simulink model "tanhModAmpModu"  (R2022a)
settings: Solver=VariableStepAuto  StartTime=0.0  StopTime=50  RelTol=1e-3
values from neighbouring files (symbols this model uses):
  bar_amp = 0.4    [setup_runAmpModu.m]
  delta_gsm = -0.025    [setup_runAmpModu.m]
  dfm1 = 0.0    (= 0)    [setup_run.m]    (also in setup_runAmpModu.m)
  dfm1s = 0.0    (= 0)    [setup_runAmpModu.m]
  dfm2 = 0.0    (= 0)    [setup_run.m]    (also in setup_runAmpModu.m)
  dsm1 = -0.5    [setup_run.m]    (also in setup_runAmpModu.m)
  dsm1s = -0.5    [setup_runAmpModu.m]
  dsm2 = -0.5    [setup_run.m]    (also in setup_runAmpModu.m)
  dsp1 = 0.5    [setup_run.m]    (also in setup_runAmpModu.m)
  dsp1s = 0.5    [setup_runAmpModu.m]
  dsp2 = 0.5    [setup_run.m]    (also in setup_runAmpModu.m)
  dup1 = -0.5    [setup_run.m]    (also in setup_runAmpModu.m)
  dup1s = -0.5    [setup_runAmpModu.m]
  dup2 = -0.5    [setup_run.m]    (also in setup_runAmpModu.m)
  gfm1 = -2.0+0.01    (= -1.99)    [setup_run.m]    (also in setup_runAmpModu.m)
  gfm1s = -2.0+0.01    (= -1.99)    [setup_runAmpModu.m]
  gfm2 = -2.0-0.01    (= -2.01)    [setup_run.m]    (also in setup_runAmpModu.m)
  gsm0 = -3.0    (= -3)    [setup_runAmpModu.m]
  gsm1s = -1.0+0.01    (= -0.99)    [setup_runAmpModu.m]
  gsp1 = 6.0-0.01    (= 5.99)    [setup_run.m]    (also in setup_runAmpModu.m = 6.99)
  gsp1s = 4.0-0.01    (= 3.99)    [setup_runAmpModu.m]
  gsp2 = 6.0+0.01    (= 6.01)    [setup_run.m]    (also in setup_runAmpModu.m = 7.01)
  gsyn12 = -0.2    [setup_run.m]    (also in setup_runAmpModu.m)
  gsyn21 = -0.2    [setup_run.m]    (also in setup_runAmpModu.m)
  gup1 = 5.0-0.01    (= 4.99)    [setup_run.m]    (also in setup_runAmpModu.m)
  gup1s = 1.0-0.01    (= 0.99)    [setup_runAmpModu.m]
  gup2 = 5.0+0.01    (= 5.01)    [setup_run.m]    (also in setup_runAmpModu.m)
  Iapp1 = -1.0    (= -1)    [setup_run.m]    (also in setup_runAmpModu.m = -1.05)
  Iapp1s = -0.05    [setup_runAmpModu.m]
  Iapp2 = -1.0    (= -1)    [setup_run.m]    (also in setup_runAmpModu.m = -0.95)
  max_torque = 10.0    (= 10)    [setup_run.m]    (also in setup_runAmpModu.m)
  noise_pwr = 0.0    (= 0)    [setup_runAmpModu.m]
  rflx_g = 0.0    (= 0)    [setup_run.m]    (also in setup_runAmpModu.m = 0.1)
undefined symbols (not defined in the file or in its folder): X, Y, Z
libraries: sm_lib x6, nesl_utility x3, simulink x3
settings Model: Creator=alessiofranci  LastModifiedBy=chris

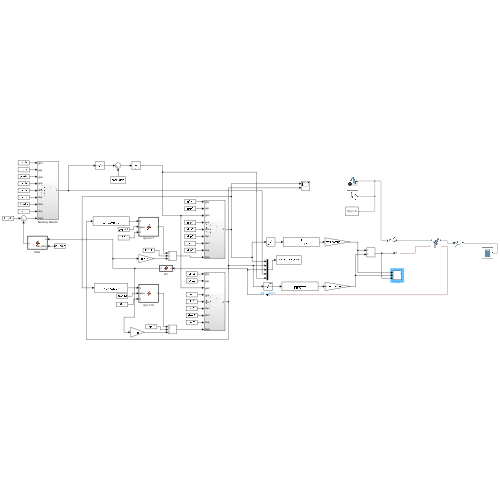
[thumbnail: Simulink's stored preview of the top-level diagram]
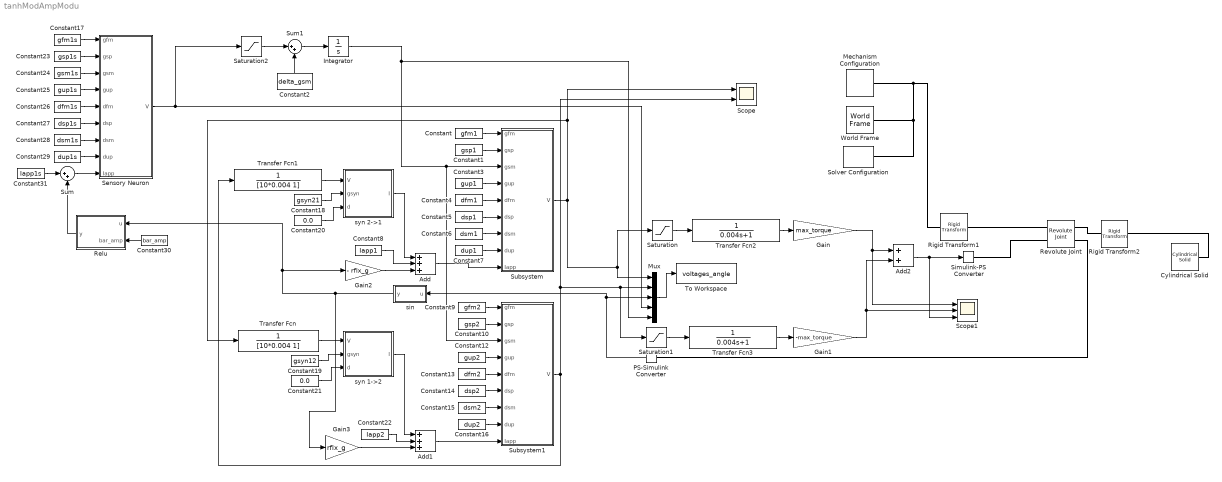
== system tanhModAmpModu ==
  Add : Sum  Inputs=+++
  Add1 : Sum  Inputs=+++
  Add2 : Sum
  Constant : Constant  Value=gfm1
  Constant1 : Constant  Value=gsp1
  Constant10 : Constant  Value=gsp2
  Constant12 : Constant  Value=gup2
  Constant13 : Constant  Value=dfm2
  Constant14 : Constant  Value=dsp2
  Constant15 : Constant  Value=dsm2
  Constant16 : Constant  Value=dup2
  Constant17 : Constant  Value=gfm1s
  Constant18 : Constant  Value=gsyn21
  Constant19 : Constant  Value=gsyn12
  Constant2 : Constant  Value=delta_gsm
  Constant20 : Constant  Value=0.0
  Constant21 : Constant  Value=0.0
  Constant22 : Constant  Value=Iapp2
  Constant23 : Constant  Value=gsp1s
  Constant24 : Constant  Value=gsm1s
  Constant25 : Constant  Value=gup1s
  Constant26 : Constant  Value=dfm1s
  Constant27 : Constant  Value=dsp1s
  Constant28 : Constant  Value=dsm1s
  Constant29 : Constant  Value=dup1s
  Constant3 : Constant  Value=gup1
  Constant30 : Constant  Value=bar_amp
  Constant31 : Constant  Value=Iapp1s
  Constant4 : Constant  Value=dfm1
  Constant5 : Constant  Value=dsp1
  Constant6 : Constant  Value=dsm1
  Constant7 : Constant  Value=dup1
  Constant8 : Constant  Value=Iapp1
  Constant9 : Constant  Value=gfm2
  Cylindrical Solid : sm_lib/Body Elements/Cylindrical Solid  GraphicAmbientColor=[0.15 0.15 0.15 1.0]  BasedOnType=Density  CenterOfMass=[0 0 0]  CenterOfMassUnits=m  GraphicDiffuseColor=[0.5 0.5 0.5]  CylinderLength=bar_length  CylinderLengthUnits=m  CylinderRadius=0.05  CylinderRadiusUnits=m  Density=1000  DensityUnits=kg/m^3  DoExposeReferenceFrame=on  GraphicEmissiveColor=[0.0 0.0 0.0 1.0]  ExportEntireGeometry=off  SerializedFrames=<Frames/>  MarkerShape=Sphere  MarkerSize=10  GraphicType=FromGeometry  InertiaType=CalculateFromGeometry  Mass=1  MassUnits=kg  MomentsOfInertia=[1 1 1]  MomentsOfInertiaUnits=kg*m^2  GraphicOpacity=1.0  ProductsOfInertia=[0 0 0]  ProductsOfInertiaUnits=kg*m^2  GraphicShininess=75  GraphicSpecularColor=[0.5 0.5 0.5 1.0]  GraphicVisPropType=SimpleVisualProperties
  Gain : Gain  Gain=max_torque
  Gain1 : Gain  Gain=-max_torque
  Gain2 : Gain  Gain=- rflx_g
  Gain3 : Gain  Gain=rflx_g
  Integrator : Integrator  InitialCondition=gsm0
  Mechanism Configuration : sm_lib/Utilities/Mechanism Configuration  UniformGravity=Constant  GravityVector=[0 0 -9.80665]  GravityUnits=m/s^2  LinearizationDelta=0.001  JointModeTransitionNonlinearIterations=2
  Mux : Mux  Inputs=5
  PS-Simulink Converter : nesl_utility/PS-Simulink Converter  PhysicalDomain=network_engine_domain  SubClassName=ps_output  LeftPortType=input  RightPortType=output  PseudoPeriodic=off  Frequencies=[]  VectorFormat=inherit  Unit=inherit  AffineConversion=off
      settings: SourceProductBaseCode=SS,PW,VE
  Relu : MATLAB Function  TreatAsAtomicUnit=on
  Revolute Joint : sm_lib/Joints/Revolute Joint  JointMode=Normal  SenseConstraintForce=off  SenseConstraintForceX=off  SenseConstraintForceY=off  SenseConstraintForceZ=off  SenseConstraintTorque=off  SenseConstraintTorqueX=off  SenseConstraintTorqueY=off  SenseConstraintTorqueZ=off  SenseTotalForce=off  SenseTotalForceX=off  SenseTotalForceY=off  SenseTotalForceZ=off  SenseTotalTorque=off  SenseTotalTorqueX=off  SenseTotalTorqueY=off  SenseTotalTorqueZ=off  CompositeWrenchDir=FollowerOnBase  CompositeWrenchFrame=BaseFrame  EquilibriumPosition=0  EquilibriumPositionUnits=deg  SpringStiffness=0.0  SpringStiffnessUnits=N*m/deg  DampingCoefficient=0.0001  DampingCoefficientUnits=N*m/(deg/s)  TorqueActuationMode=InputTorque  MotionActuationMode=ComputedMotion  SensePosition=on  SenseVelocity=off  SenseAcceleration=off  SenseTorqueForce=off  SenseLowerLimitTorqueForce=off  SenseUpperLimitTorqueForce=off  LowerLimitSpecify=off  LowerLimitBound=-90  LowerLimitBoundUnits=deg  LowerLimitStiffness=1e4  LowerLimitStiffnessUnits=N*m/deg  LowerLimitDamping=10  LowerLimitDampingUnits=N*m/(deg/s)  LowerLimitTransitionRegionWidth=0.1  LowerLimitTransitionRegionWidthUnits=deg  UpperLimitSpecify=off  UpperLimitBound=90  UpperLimitBoundUnits=deg  UpperLimitStiffness=1e4  UpperLimitStiffnessUnits=N*m/deg  UpperLimitDamping=10  UpperLimitDampingUnits=N*m/(deg/s)  UpperLimitTransitionRegionWidth=0.1  UpperLimitTransitionRegionWidthUnits=deg  PositionTargetSpecify=on  PositionTargetPriority=High  PositionTargetValue=20  PositionTargetValueUnits=deg  VelocityTargetSpecify=off  VelocityTargetPriority=High  VelocityTargetValue=0  VelocityTargetValueUnits=deg/s
  Rigid Transform1 : sm_lib/Frames and Transforms/Rigid Transform  TranslationMethod=None  TranslationStandardOffset=0.25  TranslationLengthUnit=m  TranslationStandardAxis=+X  TranslationCartesianOffset=[0 0 0]  TranslationROffset=0  TranslationROffsetUnits=m  TranslationZOffset=0  TranslationZOffsetUnits=m  TranslationThetaOffset=0  TranslationThetaOffsetUnits=deg  RotationMethod=RotationSequence  RotationAngleUnits=deg  RotationStandardAxis=+Y  RotationAngle=90  RotationArbitraryAxis=[0 0 1]  FollAlignAxisA=+X  BaseAlignAxisA=+Y  FollAlignAxisB=+Y  BaseAlignAxisB=+Z  RotationSequenceAxes=FollowerAxes  RotationSequence=XYX  RotationSequenceAngles=[0 90 90]  RotationSequenceAnglesUnits=deg  RotationMatrix=[1 0 0; 0 1 0; 0 0 1]
  Rigid Transform2 : sm_lib/Frames and Transforms/Rigid Transform  TranslationMethod=StandardAxis  TranslationStandardOffset=.25  TranslationLengthUnit=m  TranslationStandardAxis=+X  TranslationCartesianOffset=[0 0 0]  TranslationROffset=0  TranslationROffsetUnits=m  TranslationZOffset=0  TranslationZOffsetUnits=m  TranslationThetaOffset=0  TranslationThetaOffsetUnits=deg  RotationMethod=RotationSequence  RotationAngleUnits=deg  RotationStandardAxis=+Z  RotationAngle=90  RotationArbitraryAxis=[0 0 1]  FollAlignAxisA=+X  BaseAlignAxisA=+Y  FollAlignAxisB=+Y  BaseAlignAxisB=+Z  RotationSequenceAxes=FollowerAxes  RotationSequence=XYX  RotationSequenceAngles=[0 90 0]  RotationSequenceAnglesUnits=deg  RotationMatrix=[1 0 0; 0 1 0; 0 0 1]
  Saturation : Saturate  UpperLimit=1.0  LowerLimit=0.0
  Saturation1 : Saturate  UpperLimit=1.0  LowerLimit=0.0
  Saturation2 : Saturate  UpperLimit=1.0  LowerLimit=0.0
  Scope : Scope  NumInputPorts=2
  Scope1 : Scope  NumInputPorts=3
  Sensory Neuron : Subsystem
  Simulink-PS Converter : nesl_utility/Simulink-PS Converter  PhysicalDomain=network_engine_domain  SubClassName=ps_input  LeftPortType=input  RightPortType=output  PseudoPeriodic=off  Frequencies=[]  NoiseDistribution=none  NoiseParameters=[]  Unit=1  AffineConversion=off  FilteringAndDerivatives=provide  SimscapeFilterOrder=1  InputFilterTimeConstant=0.001  UdotUserProvided=0
      settings: SourceProductBaseCode=SS,PW,VE
  Solver Configuration : nesl_utility/Solver Configuration  PhysicalDomain=network_engine_domain  SubClassName=solver  LeftPortType=input  RightPortType=generic  Tones=[]  Harmonics=[]  SimulateNoise=off  Profile=off  UseLocalSampling=off  EnableSwitchedLinearOptims=on  FrequencyDomain=off  UseCCode=off  RelTol=0.001  AbsTol=1e-06  MinStep=1e-09  ToWorkspace=off  RevertToSquareIcSolve=off  NumHomotopyIterations=100  PhasorMode=off  PhasorModeNumHarmonics=1  IndexReductionMethod=DerivativeReplacement  DoDC=off  ResidualTolerance=1e-09  UseLocalSolver=off  LocalSolverChoice=NE_BACKWARD_EULER_ADVANCER  LocalSolverSampleTime=0.001  DoFixedCost=off  MaxNonlinIter=3  MaxModeIter=2  ComputeImpulses=off  ImpulseIterations=2  LinearAlgebra=auto  LinearAlgebraNumThread=0  EquationFormulation=NE_TIME_EF  DelaysMemoryBudget=1024  AutomaticFiltering=on  FilteringTimeConstant=0.001  PartitionStorageMethod=AS_NEEDED  PartitionMemoryBudget=1024  PartitionMethod=ROBUST
      settings: SourceProductBaseCode=SS,PW,VE
  Subsystem : Subsystem
  Subsystem1 : Subsystem
  Sum : Sum  Inputs=|++
  Sum1 : Sum  Inputs=|++
  To Workspace : ToWorkspace  VariableName=voltages_angle  SaveFormat=Structure With Time  SampleTime=-1
  Transfer Fcn : TransferFcn  Denominator=[10*0.004 1]
  Transfer Fcn1 : TransferFcn  Denominator=[10*0.004 1]
  Transfer Fcn2 : TransferFcn  Denominator=[0.004 1]
  Transfer Fcn3 : TransferFcn  Denominator=[0.004 1]
  World Frame : sm_lib/Frames and Transforms/World Frame
  sin : MATLAB Function  TreatAsAtomicUnit=on
  syn 1->2 : MATLAB Function  TreatAsAtomicUnit=on
  syn 2->1 : MATLAB Function  TreatAsAtomicUnit=on
  wires:
  Constant5/1 -> Subsystem/6(dsp)
  Constant3/1 -> Subsystem/4(gup)
  Constant1/1 -> Subsystem/2(gsp)
  Constant8/1 -> Add/2
  Saturation1/1 -> Transfer Fcn3/1
  syn 1->2/1(I) -> Add1/1
  Subsystem1/1(V) -> Scope/2, Saturation1/1, Mux/2, Transfer Fcn1/1
  Constant15/1 -> Subsystem1/7(dsm)
  syn 2->1/1(I) -> Add/1
  Constant16/1 -> Subsystem1/8(dup)
  Constant22/1 -> Add1/2
  Add1/1 -> Subsystem1/9(Iapp)
  Gain2/1 -> Add/3
  Constant/1 -> Subsystem/1(gfm)
  Add/1 -> Subsystem/9(Iapp)
  Subsystem/1(V) -> Saturation/1, Mux/1, Scope/1, Transfer Fcn/1
  Constant18/1 -> syn 2->1/2(gsyn)
  Constant7/1 -> Subsystem/8(dup)
  Mux/1 -> To Workspace/1
  Constant20/1 -> syn 2->1/3(d)
  Constant10/1 -> Subsystem1/2(gsp)
  Gain1/1 -> Add2/2, Scope1/2
  Constant13/1 -> Subsystem1/5(dfm)
  PS-Simulink Converter/1 -> sin/1(u), Mux/3
  Transfer Fcn1/1 -> syn 2->1/1(V)
  Gain/1 -> Add2/1, Scope1/1
  Constant19/1 -> syn 1->2/2(gsyn)
  Transfer Fcn/1 -> syn 1->2/1(V)
  Constant21/1 -> syn 1->2/3(d)
  Constant4/1 -> Subsystem/5(dfm)
  Constant14/1 -> Subsystem1/6(dsp)
  Constant12/1 -> Subsystem1/4(gup)
  Constant6/1 -> Subsystem/7(dsm)
  Constant9/1 -> Subsystem1/1(gfm)
  Gain3/1 -> Add1/3
  Constant23/1 -> Sensory Neuron/2(gsp)
  Constant29/1 -> Sensory Neuron/8(dup)
  Constant27/1 -> Sensory Neuron/6(dsp)
  Constant25/1 -> Sensory Neuron/4(gup)
  Constant24/1 -> Sensory Neuron/3(gsm)
  Constant17/1 -> Sensory Neuron/1(gfm)
  Constant28/1 -> Sensory Neuron/7(dsm)
  Constant26/1 -> Sensory Neuron/5(dfm)
  Sensory Neuron/1(V) -> Saturation2/1, Mux/4
  sin/1(y) -> Gain2/1, Relu/1(u), Gain3/1
  Constant30/1 -> Relu/2(bar_amp)
  Constant31/1 -> Sum/1
  Sum/1 -> Sensory Neuron/9(Iapp)
  Relu/1(y) -> Sum/2
  Sum1/1 -> Integrator/1
  Constant2/1 -> Sum1/2
  Saturation2/1 -> Sum1/1
  Integrator/1 -> Subsystem1/3(gsm), Subsystem/3(gsm), Mux/5
  Add2/1 -> Scope1/3, Simulink-PS Converter/1
  Saturation/1 -> Transfer Fcn2/1
  Transfer Fcn2/1 -> Gain/1
  Transfer Fcn3/1 -> Gain1/1
  connections:
  Solver Configuration/RConn1 -- World Frame/RConn1 -- Mechanism Configuration/RConn1 -- Rigid Transform1/LConn1
  Rigid Transform1/RConn1 -- Revolute Joint/LConn1
  Rigid Transform2/LConn1 -- Revolute Joint/RConn1
  Simulink-PS Converter/RConn1 -- Revolute Joint/LConn2
  Rigid Transform2/RConn1 -- Cylindrical Solid/RConn1
  Revolute Joint/RConn2 -- PS-Simulink Converter/LConn1

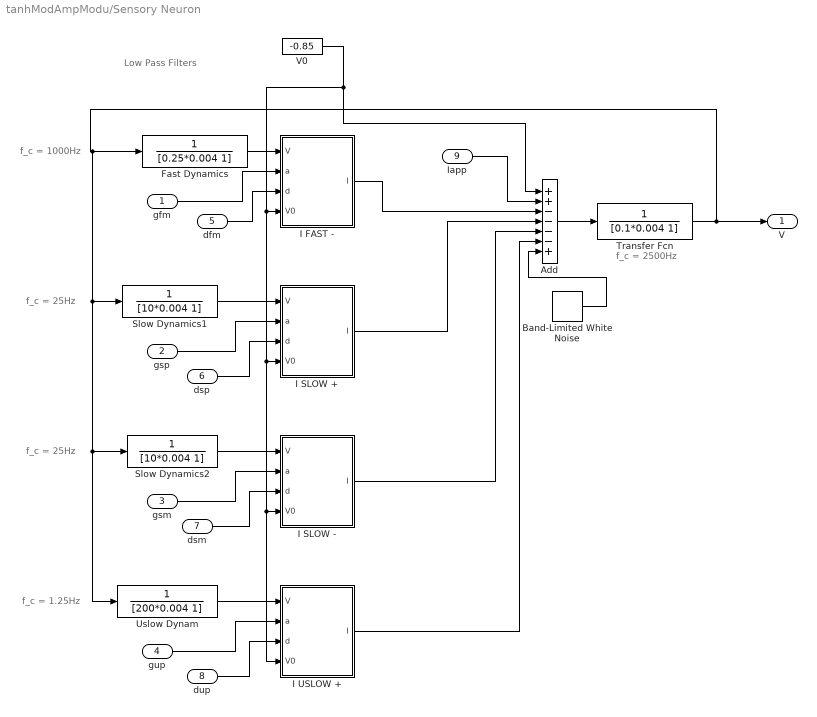
== system tanhModAmpModu/Sensory Neuron ==
  note: f_c = 2500Hz
  note: f_c = 1.25Hz
  note: f_c = 25Hz
  note: f_c = 1000Hz
  note: Low Pass Filters
  note: f_c = 25Hz
  gfm : Inport
  gsp : Inport  Port=2
  gsm : Inport  Port=3
  gup : Inport  Port=4
  dfm : Inport  Port=5
  dsp : Inport  Port=6
  dsm : Inport  Port=7
  dup : Inport  Port=8
  Iapp : Inport  Port=9
  Add : Sum  Inputs=++----+
  Band-Limited White Noise : simulink/Sources/Band-Limited White Noise  Cov=[0.0]  Ts=0.1  seed=[23341]
  Fast Dynamics : TransferFcn  Denominator=[0.25*0.004 1]
  I FAST - : MATLAB Function  TreatAsAtomicUnit=on
  I SLOW + : MATLAB Function  TreatAsAtomicUnit=on
  I SLOW - : MATLAB Function  TreatAsAtomicUnit=on
  I USLOW + : MATLAB Function  TreatAsAtomicUnit=on
  Slow Dynamics1 : TransferFcn  Denominator=[10*0.004 1]
  Slow Dynamics2 : TransferFcn  Denominator=[10*0.004 1]
  Transfer Fcn : TransferFcn  Denominator=[0.1*0.004 1]
  Uslow Dynam : TransferFcn  Denominator=[200*0.004 1]
  V0 : Constant  Value=-0.85
  V : Outport
  wires:
  dup/1 -> I USLOW +/3(d)
  gsm/1 -> I SLOW -/2(a)
  dsm/1 -> I SLOW -/3(d)
  gup/1 -> I USLOW +/2(a)
  Iapp/1 -> Add/2
  Uslow Dynam/1 -> I USLOW +/1(V)
  Add/1 -> Transfer Fcn/1
  Slow Dynamics1/1 -> I SLOW +/1(V)
  Slow Dynamics2/1 -> I SLOW -/1(V)
  I FAST -/1(I) -> Add/3
  I USLOW +/1(I) -> Add/6
  V0/1 -> I USLOW +/4(V0), I SLOW -/4(V0), I SLOW +/4(V0), I FAST -/4(V0), Add/1
  dsp/1 -> I SLOW +/3(d)
  gsp/1 -> I SLOW +/2(a)
  dfm/1 -> I FAST -/3(d)
  gfm/1 -> I FAST -/2(a)
  Fast Dynamics/1 -> I FAST -/1(V)
  I SLOW -/1(I) -> Add/5
  Transfer Fcn/1 -> V/1, Uslow Dynam/1, Slow Dynamics2/1, Slow Dynamics1/1, Fast Dynamics/1
  I SLOW +/1(I) -> Add/4
  Band-Limited White Noise/1 -> Add/7

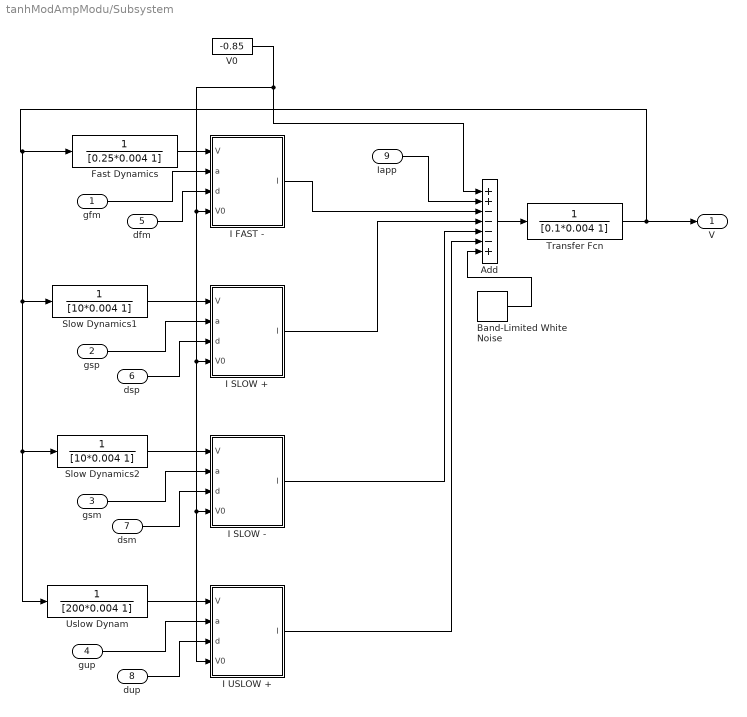
== system tanhModAmpModu/Subsystem ==
  gfm : Inport
  gsp : Inport  Port=2
  gsm : Inport  Port=3
  gup : Inport  Port=4
  dfm : Inport  Port=5
  dsp : Inport  Port=6
  dsm : Inport  Port=7
  dup : Inport  Port=8
  Iapp : Inport  Port=9
  Add : Sum  Inputs=++----+
  Band-Limited White Noise : simulink/Sources/Band-Limited White Noise  Cov=noise_pwr  Ts=0.01  seed=[23341]
  Fast Dynamics : TransferFcn  Denominator=[0.25*0.004 1]
  I FAST - : MATLAB Function  TreatAsAtomicUnit=on
  I SLOW + : MATLAB Function  TreatAsAtomicUnit=on
  I SLOW - : MATLAB Function  TreatAsAtomicUnit=on
  I USLOW + : MATLAB Function  TreatAsAtomicUnit=on
  Slow Dynamics1 : TransferFcn  Denominator=[10*0.004 1]
  Slow Dynamics2 : TransferFcn  Denominator=[10*0.004 1]
  Transfer Fcn : TransferFcn  Denominator=[0.1*0.004 1]
  Uslow Dynam : TransferFcn  Denominator=[200*0.004 1]
  V0 : Constant  Value=-0.85
  V : Outport
  wires:
  dup/1 -> I USLOW +/3(d)
  gsm/1 -> I SLOW -/2(a)
  dsm/1 -> I SLOW -/3(d)
  gup/1 -> I USLOW +/2(a)
  Iapp/1 -> Add/2
  Uslow Dynam/1 -> I USLOW +/1(V)
  Add/1 -> Transfer Fcn/1
  Slow Dynamics1/1 -> I SLOW +/1(V)
  Slow Dynamics2/1 -> I SLOW -/1(V)
  I FAST -/1(I) -> Add/3
  I USLOW +/1(I) -> Add/6
  V0/1 -> I USLOW +/4(V0), I SLOW -/4(V0), I SLOW +/4(V0), I FAST -/4(V0), Add/1
  dsp/1 -> I SLOW +/3(d)
  gsp/1 -> I SLOW +/2(a)
  dfm/1 -> I FAST -/3(d)
  gfm/1 -> I FAST -/2(a)
  Fast Dynamics/1 -> I FAST -/1(V)
  I SLOW -/1(I) -> Add/5
  Transfer Fcn/1 -> V/1, Uslow Dynam/1, Slow Dynamics2/1, Slow Dynamics1/1, Fast Dynamics/1
  I SLOW +/1(I) -> Add/4
  Band-Limited White Noise/1 -> Add/7

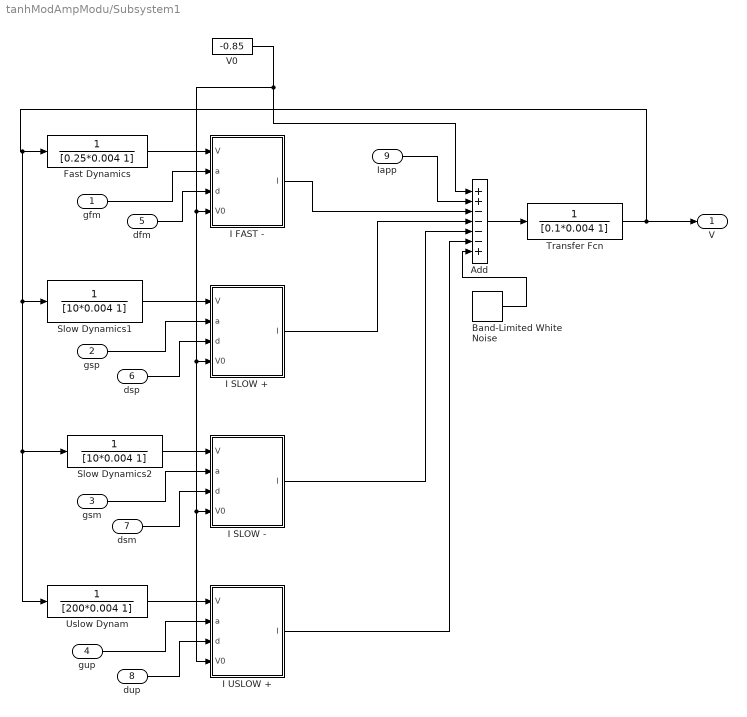
== system tanhModAmpModu/Subsystem1 ==
  gfm : Inport
  gsp : Inport  Port=2
  gsm : Inport  Port=3
  gup : Inport  Port=4
  dfm : Inport  Port=5
  dsp : Inport  Port=6
  dsm : Inport  Port=7
  dup : Inport  Port=8
  Iapp : Inport  Port=9
  Add : Sum  Inputs=++----+
  Band-Limited White Noise : simulink/Sources/Band-Limited White Noise  Cov=[noise_pwr]  Ts=0.01  seed=[23341]
  Fast Dynamics : TransferFcn  Denominator=[0.25*0.004 1]
  I FAST - : MATLAB Function  TreatAsAtomicUnit=on
  I SLOW + : MATLAB Function  TreatAsAtomicUnit=on
  I SLOW - : MATLAB Function  TreatAsAtomicUnit=on
  I USLOW + : MATLAB Function  TreatAsAtomicUnit=on
  Slow Dynamics1 : TransferFcn  Denominator=[10*0.004 1]
  Slow Dynamics2 : TransferFcn  Denominator=[10*0.004 1]
  Transfer Fcn : TransferFcn  Denominator=[0.1*0.004 1]
  Uslow Dynam : TransferFcn  Denominator=[200*0.004 1]
  V0 : Constant  Value=-0.85
  V : Outport
  wires:
  dup/1 -> I USLOW +/3(d)
  gsm/1 -> I SLOW -/2(a)
  dsm/1 -> I SLOW -/3(d)
  gup/1 -> I USLOW +/2(a)
  Iapp/1 -> Add/2
  Uslow Dynam/1 -> I USLOW +/1(V)
  Add/1 -> Transfer Fcn/1
  Slow Dynamics1/1 -> I SLOW +/1(V)
  Slow Dynamics2/1 -> I SLOW -/1(V)
  I FAST -/1(I) -> Add/3
  I USLOW +/1(I) -> Add/6
  V0/1 -> I USLOW +/4(V0), I SLOW -/4(V0), I SLOW +/4(V0), I FAST -/4(V0), Add/1
  dsp/1 -> I SLOW +/3(d)
  gsp/1 -> I SLOW +/2(a)
  dfm/1 -> I FAST -/3(d)
  gfm/1 -> I FAST -/2(a)
  Fast Dynamics/1 -> I FAST -/1(V)
  I SLOW -/1(I) -> Add/5
  Transfer Fcn/1 -> V/1, Uslow Dynam/1, Slow Dynamics2/1, Slow Dynamics1/1, Fast Dynamics/1
  I SLOW +/1(I) -> Add/4
  Band-Limited White Noise/1 -> Add/7

== matlab function tanhModAmpModu/Subsystem/I SLOW + ==
  data: V input; I output; a input; d input; V0 input
function I = fcn(V,a,d,V0)

I = a*(tanh(V-d)-tanh(V0-d));

== matlab function tanhModAmpModu/sin ==
  data: u input; y output
function y = fcn(u)

y = sin(u);

== matlab function tanhModAmpModu/Sensory Neuron/I FAST - ==
  data: V input; I output; a input; d input; V0 input
function I = fcn(V,a,d,V0)

I = a*(tanh(V-d)-tanh(V0-d));

== matlab function tanhModAmpModu/Sensory Neuron/I SLOW + ==
  data: V input; I output; a input; d input; V0 input
function I = fcn(V,a,d,V0)

I = a*(tanh(V-d)-tanh(V0-d));

== matlab function tanhModAmpModu/Sensory Neuron/I SLOW - ==
  data: V input; I output; a input; d input; V0 input
function I = fcn(V,a,d,V0)

I = a*(tanh(V-d)-tanh(V0-d));

== matlab function tanhModAmpModu/Sensory Neuron/I USLOW + ==
  data: V input; I output; a input; d input; V0 input
function I = fcn(V,a,d,V0)

I = a*(tanh(V-d)-tanh(V0-d));

== matlab function tanhModAmpModu/Relu ==
  data: u input; y output; bar_amp input
function y = fcn(u,bar_amp)

y = max(0,u-sin(bar_amp));

== matlab function tanhModAmpModu/Subsystem/I FAST - ==
  data: V input; I output; a input; d input; V0 input
function I = fcn(V,a,d,V0)

I = a*(tanh(V-d)-tanh(V0-d));

== matlab function tanhModAmpModu/Subsystem/I SLOW - ==
  data: V input; I output; a input; d input; V0 input
function I = fcn(V,a,d,V0)

I = a*(tanh(V-d)-tanh(V0-d));

== matlab function tanhModAmpModu/Subsystem/I USLOW + ==
  data: V input; I output; a input; d input; V0 input
function I = fcn(V,a,d,V0)

I = a*(tanh(V-d)-tanh(V0-d));

== matlab function tanhModAmpModu/Subsystem1/I FAST - ==
  data: V input; I output; a input; d input; V0 input
function I = fcn(V,a,d,V0)

I = a*(tanh(V-d)-tanh(V0-d));

== matlab function tanhModAmpModu/Subsystem1/I SLOW + ==
  data: V input; I output; a input; d input; V0 input
function I = fcn(V,a,d,V0)

I = a*(tanh(V-d)-tanh(V0-d));

== matlab function tanhModAmpModu/Subsystem1/I SLOW - ==
  data: V input; I output; a input; d input; V0 input
function I = fcn(V,a,d,V0)

I = a*(tanh(V-d)-tanh(V0-d));

== matlab function tanhModAmpModu/Subsystem1/I USLOW + ==
  data: V input; I output; a input; d input; V0 input
function I = fcn(V,a,d,V0)

I = a*(tanh(V-d)-tanh(V0-d));

== matlab function tanhModAmpModu/syn 1->2 ==
  data: V input; I output; gsyn input; d input
function I = fcn(V,gsyn,d)

I = gsyn*(tanh(2*(V-d))+1)/2;

== matlab function tanhModAmpModu/syn 2->1 ==
  data: V input; I output; gsyn input; d input
function I = fcn(V,gsyn,d)

I = gsyn*(tanh(2*(V-d))+1)/2;
